simulink model "D_20231120_Modell_Inbetriebnahme_BreakOutBox_Jetson"  (R2022b)
(part 6 of 8)

  CAN Unpack94/16 -> Bus Creator94/7  "CAN ID"
  CAN Unpack94/17 -> Bus Creator94/8  "Timestamp"
  Bus Creator94/1 -> Bus Creator1/94  "Data_093"
  CAN Unpack94/1 -> Bus Creator94/1  "AZ_Winkel"
  CAN Unpack95/3 -> Terminator840/1
  CAN Unpack95/2 -> Bus Creator95/2  "EL_Angle"
  CAN Unpack95/13 -> Terminator847/1
  CAN Unpack95/7 -> Terminator844/1
  CAN Unpack95/12 -> Bus Creator95/5  "Range"
  CAN Unpack95/10 -> Bus Creator95/3  "Mode_Signal"
  CAN Unpack95/4 -> Terminator841/1
  CAN Unpack95/5 -> Terminator842/1
  CAN Unpack95/8 -> Terminator845/1
  CAN Unpack95/11 -> Bus Creator95/4  "RCS"
  CAN Unpack95/14 -> Terminator848/1
  CAN Unpack95/15 -> Bus Creator95/6  "Speed_Radial"
  CAN Unpack95/9 -> Terminator846/1
  CAN Unpack95/6 -> Terminator843/1
  CAN Unpack95/16 -> Bus Creator95/7  "CAN ID"
  CAN Unpack95/17 -> Bus Creator95/8  "Timestamp"
  Bus Creator95/1 -> Bus Creator1/95  "Data_094"
  CAN Unpack95/1 -> Bus Creator95/1  "AZ_Winkel"
  CAN Unpack96/3 -> Terminator849/1
  CAN Unpack96/2 -> Bus Creator96/2  "EL_Angle"
  CAN Unpack96/13 -> Terminator856/1
  CAN Unpack96/7 -> Terminator853/1
  CAN Unpack96/12 -> Bus Creator96/5  "Range"
  CAN Unpack96/10 -> Bus Creator96/3  "Mode_Signal"
  CAN Unpack96/4 -> Terminator850/1
  CAN Unpack96/5 -> Terminator851/1
  CAN Unpack96/8 -> Terminator854/1
  CAN Unpack96/11 -> Bus Creator96/4  "RCS"
  CAN Unpack96/14 -> Terminator857/1
  CAN Unpack96/15 -> Bus Creator96/6  "Speed_Radial"
  CAN Unpack96/9 -> Terminator855/1
  CAN Unpack96/6 -> Terminator852/1
  CAN Unpack96/16 -> Bus Creator96/7  "CAN ID"
  CAN Unpack96/17 -> Bus Creator96/8  "Timestamp"
  Bus Creator96/1 -> Bus Creator1/96  "Data_095"
  CAN Unpack96/1 -> Bus Creator96/1  "AZ_Winkel"
  CAN Unpack97/3 -> Terminator858/1
  CAN Unpack97/2 -> Bus Creator97/2  "EL_Angle"
  CAN Unpack97/13 -> Terminator865/1
  CAN Unpack97/7 -> Terminator862/1
  CAN Unpack97/12 -> Bus Creator97/5  "Range"
  CAN Unpack97/10 -> Bus Creator97/3  "Mode_Signal"
  CAN Unpack97/4 -> Terminator859/1
  CAN Unpack97/5 -> Terminator860/1
  CAN Unpack97/8 -> Terminator863/1
  CAN Unpack97/11 -> Bus Creator97/4  "RCS"
  CAN Unpack97/14 -> Terminator866/1
  CAN Unpack97/15 -> Bus Creator97/6  "Speed_Radial"
  CAN Unpack97/9 -> Terminator864/1
  CAN Unpack97/6 -> Terminator861/1
  CAN Unpack97/16 -> Bus Creator97/7  "CAN ID"
  CAN Unpack97/17 -> Bus Creator97/8  "Timestamp"
  Bus Creator97/1 -> Bus Creator1/97  "Data_096"
  CAN Unpack97/1 -> Bus Creator97/1  "AZ_Winkel"
  CAN Unpack98/3 -> Terminator867/1
  CAN Unpack98/2 -> Bus Creator98/2  "EL_Angle"
  CAN Unpack98/13 -> Terminator874/1
  CAN Unpack98/7 -> Terminator871/1
  CAN Unpack98/12 -> Bus Creator98/5  "Range"
  CAN Unpack98/10 -> Bus Creator98/3  "Mode_Signal"
  CAN Unpack98/4 -> Terminator868/1
  CAN Unpack98/5 -> Terminator869/1
  CAN Unpack98/8 -> Terminator872/1
  CAN Unpack98/11 -> Bus Creator98/4  "RCS"
  CAN Unpack98/14 -> Terminator875/1
  CAN Unpack98/15 -> Bus Creator98/6  "Speed_Radial"
  CAN Unpack98/9 -> Terminator873/1
  CAN Unpack98/6 -> Terminator870/1
  CAN Unpack98/16 -> Bus Creator98/7  "CAN ID"
  CAN Unpack98/17 -> Bus Creator98/8  "Timestamp"
  Bus Creator98/1 -> Bus Creator1/98  "Data_097"
  CAN Unpack98/1 -> Bus Creator98/1  "AZ_Winkel"
  CAN Unpack99/3 -> Terminator876/1
  CAN Unpack99/2 -> Bus Creator99/2  "EL_Angle"
  CAN Unpack99/13 -> Terminator883/1
  CAN Unpack99/7 -> Terminator880/1
  CAN Unpack99/12 -> Bus Creator99/5  "Range"
  CAN Unpack99/10 -> Bus Creator99/3  "Mode_Signal"
  CAN Unpack99/4 -> Terminator877/1
  CAN Unpack99/5 -> Terminator878/1
  CAN Unpack99/8 -> Terminator881/1
  CAN Unpack99/11 -> Bus Creator99/4  "RCS"
  CAN Unpack99/14 -> Terminator884/1
  CAN Unpack99/15 -> Bus Creator99/6  "Speed_Radial"
  CAN Unpack99/9 -> Terminator882/1
  CAN Unpack99/6 -> Terminator879/1
  CAN Unpack99/16 -> Bus Creator99/7  "CAN ID"
  CAN Unpack99/17 -> Bus Creator99/8  "Timestamp"
  Bus Creator99/1 -> Bus Creator1/99  "Data_098"
  CAN Unpack99/1 -> Bus Creator99/1  "AZ_Winkel"
  CAN Unpack100/3 -> Terminator885/1
  CAN Unpack100/2 -> Bus Creator100/2  "EL_Angle"
  CAN Unpack100/13 -> Terminator892/1
  CAN Unpack100/7 -> Terminator889/1
  CAN Unpack100/12 -> Bus Creator100/5  "Range"
  CAN Unpack100/10 -> Bus Creator100/3  "Mode_Signal"
  CAN Unpack100/4 -> Terminator886/1
  CAN Unpack100/5 -> Terminator887/1
  CAN Unpack100/8 -> Terminator890/1
  CAN Unpack100/11 -> Bus Creator100/4  "RCS"
  CAN Unpack100/14 -> Terminator893/1
  CAN Unpack100/15 -> Bus Creator100/6  "Speed_Radial"
  CAN Unpack100/9 -> Terminator891/1
  CAN Unpack100/6 -> Terminator888/1
  CAN Unpack100/16 -> Bus Creator100/7  "CAN ID"
  CAN Unpack100/17 -> Bus Creator100/8  "Timestamp"
  Bus Creator100/1 -> Bus Creator1/100  "Data_099"
  CAN Unpack100/1 -> Bus Creator100/1  "AZ_Winkel"
  CAN Unpack101/3 -> Terminator894/1
  CAN Unpack101/2 -> Bus Creator101/2  "EL_Angle"
  CAN Unpack101/13 -> Terminator901/1
  CAN Unpack101/7 -> Terminator898/1
  CAN Unpack101/12 -> Bus Creator101/5  "Range"
  CAN Unpack101/10 -> Bus Creator101/3  "Mode_Signal"
  CAN Unpack101/4 -> Terminator895/1
  CAN Unpack101/5 -> Terminator896/1
  CAN Unpack101/8 -> Terminator899/1
  CAN Unpack101/11 -> Bus Creator101/4  "RCS"
  CAN Unpack101/14 -> Terminator902/1
  CAN Unpack101/15 -> Bus Creator101/6  "Speed_Radial"
  CAN Unpack101/9 -> Terminator900/1
  CAN Unpack101/6 -> Terminator897/1
  CAN Unpack101/16 -> Bus Creator101/7  "CAN ID"
  CAN Unpack101/17 -> Bus Creator101/8  "Timestamp"
  Bus Creator101/1 -> Bus Creator1/101  "Data_100"
  CAN Unpack101/1 -> Bus Creator101/1  "AZ_Winkel"
  CAN Unpack102/3 -> Terminator903/1
  CAN Unpack102/2 -> Bus Creator102/2  "EL_Angle"
  CAN Unpack102/13 -> Terminator910/1
  CAN Unpack102/7 -> Terminator907/1
  CAN Unpack102/12 -> Bus Creator102/5  "Range"
  CAN Unpack102/10 -> Bus Creator102/3  "Mode_Signal"
  CAN Unpack102/4 -> Terminator904/1
  CAN Unpack102/5 -> Terminator905/1
  CAN Unpack102/8 -> Terminator908/1
  CAN Unpack102/11 -> Bus Creator102/4  "RCS"
  CAN Unpack102/14 -> Terminator911/1
  CAN Unpack102/15 -> Bus Creator102/6  "Speed_Radial"
  CAN Unpack102/9 -> Terminator909/1
  CAN Unpack102/6 -> Terminator906/1
  CAN Unpack102/16 -> Bus Creator102/7  "CAN ID"
  CAN Unpack102/17 -> Bus Creator102/8  "Timestamp"
  Bus Creator102/1 -> Bus Creator1/102  "Data_101"
  CAN Unpack102/1 -> Bus Creator102/1  "AZ_Winkel"
  CAN Unpack103/3 -> Terminator912/1
  CAN Unpack103/2 -> Bus Creator103/2  "EL_Angle"
  CAN Unpack103/13 -> Terminator919/1
  CAN Unpack103/7 -> Terminator916/1
  CAN Unpack103/12 -> Bus Creator103/5  "Range"
  CAN Unpack103/10 -> Bus Creator103/3  "Mode_Signal"
  CAN Unpack103/4 -> Terminator913/1
  CAN Unpack103/5 -> Terminator914/1
  CAN Unpack103/8 -> Terminator917/1
  CAN Unpack103/11 -> Bus Creator103/4  "RCS"
  CAN Unpack103/14 -> Terminator920/1
  CAN Unpack103/15 -> Bus Creator103/6  "Speed_Radial"
  CAN Unpack103/9 -> Terminator918/1
  CAN Unpack103/6 -> Terminator915/1
  CAN Unpack103/16 -> Bus Creator103/7  "CAN ID"
  CAN Unpack103/17 -> Bus Creator103/8  "Timestamp"
  Bus Creator103/1 -> Bus Creator1/103  "Data_102"
  CAN Unpack103/1 -> Bus Creator103/1  "AZ_Winkel"
  CAN Unpack104/3 -> Terminator921/1
  CAN Unpack104/2 -> Bus Creator104/2  "EL_Angle"
  CAN Unpack104/13 -> Terminator928/1
  CAN Unpack104/7 -> Terminator925/1
  CAN Unpack104/12 -> Bus Creator104/5  "Range"
  CAN Unpack104/10 -> Bus Creator104/3  "Mode_Signal"
  CAN Unpack104/4 -> Terminator922/1
  CAN Unpack104/5 -> Terminator923/1
  CAN Unpack104/8 -> Terminator926/1
  CAN Unpack104/11 -> Bus Creator104/4  "RCS"
  CAN Unpack104/14 -> Terminator929/1
  CAN Unpack104/15 -> Bus Creator104/6  "Speed_Radial"
  CAN Unpack104/9 -> Terminator927/1
  CAN Unpack104/6 -> Terminator924/1
  CAN Unpack104/16 -> Bus Creator104/7  "CAN ID"
  CAN Unpack104/17 -> Bus Creator104/8  "Timestamp"
  Bus Creator104/1 -> Bus Creator1/104  "Data_103"
  CAN Unpack104/1 -> Bus Creator104/1  "AZ_Winkel"
  CAN Unpack105/3 -> Terminator930/1
  CAN Unpack105/2 -> Bus Creator105/2  "EL_Angle"
  CAN Unpack105/13 -> Terminator937/1
  CAN Unpack105/7 -> Terminator934/1
  CAN Unpack105/12 -> Bus Creator105/5  "Range"
  CAN Unpack105/10 -> Bus Creator105/3  "Mode_Signal"
  CAN Unpack105/4 -> Terminator931/1
  CAN Unpack105/5 -> Terminator932/1
  CAN Unpack105/8 -> Terminator935/1
  CAN Unpack105/11 -> Bus Creator105/4  "RCS"
  CAN Unpack105/14 -> Terminator938/1
  CAN Unpack105/15 -> Bus Creator105/6  "Speed_Radial"
  CAN Unpack105/9 -> Terminator936/1
  CAN Unpack105/6 -> Terminator933/1
  CAN Unpack105/16 -> Bus Creator105/7  "CAN ID"
  CAN Unpack105/17 -> Bus Creator105/8  "Timestamp"
  Bus Creator105/1 -> Bus Creator1/105  "Data_104"
  CAN Unpack105/1 -> Bus Creator105/1  "AZ_Winkel"
  CAN Unpack106/3 -> Terminator939/1
  CAN Unpack106/2 -> Bus Creator106/2  "EL_Angle"
  CAN Unpack106/13 -> Terminator946/1
  CAN Unpack106/7 -> Terminator943/1
  CAN Unpack106/12 -> Bus Creator106/5  "Range"
  CAN Unpack106/10 -> Bus Creator106/3  "Mode_Signal"
  CAN Unpack106/4 -> Terminator940/1
  CAN Unpack106/5 -> Terminator941/1
  CAN Unpack106/8 -> Terminator944/1
  CAN Unpack106/11 -> Bus Creator106/4  "RCS"
  CAN Unpack106/14 -> Terminator947/1
  CAN Unpack106/15 -> Bus Creator106/6  "Speed_Radial"
  CAN Unpack106/9 -> Terminator945/1
  CAN Unpack106/6 -> Terminator942/1
  CAN Unpack106/16 -> Bus Creator106/7  "CAN ID"
  CAN Unpack106/17 -> Bus Creator106/8  "Timestamp"
  Bus Creator106/1 -> Bus Creator1/106  "Data_105"
  CAN Unpack106/1 -> Bus Creator106/1  "AZ_Winkel"
  CAN Unpack107/3 -> Terminator948/1
  CAN Unpack107/2 -> Bus Creator107/2  "EL_Angle"
  CAN Unpack107/13 -> Terminator955/1
  CAN Unpack107/7 -> Terminator952/1
  CAN Unpack107/12 -> Bus Creator107/5  "Range"
  CAN Unpack107/10 -> Bus Creator107/3  "Mode_Signal"
  CAN Unpack107/4 -> Terminator949/1
  CAN Unpack107/5 -> Terminator950/1
  CAN Unpack107/8 -> Terminator953/1
  CAN Unpack107/11 -> Bus Creator107/4  "RCS"
  CAN Unpack107/14 -> Terminator956/1
  CAN Unpack107/15 -> Bus Creator107/6  "Speed_Radial"
  CAN Unpack107/9 -> Terminator954/1
  CAN Unpack107/6 -> Terminator951/1
  CAN Unpack107/16 -> Bus Creator107/7  "CAN ID"
  CAN Unpack107/17 -> Bus Creator107/8  "Timestamp"
  Bus Creator107/1 -> Bus Creator1/107  "Data_106"
  CAN Unpack107/1 -> Bus Creator107/1  "AZ_Winkel"
  CAN Unpack108/3 -> Terminator957/1
  CAN Unpack108/2 -> Bus Creator108/2  "EL_Angle"
  CAN Unpack108/13 -> Terminator964/1
  CAN Unpack108/7 -> Terminator961/1
  CAN Unpack108/12 -> Bus Creator108/5  "Range"
  CAN Unpack108/10 -> Bus Creator108/3  "Mode_Signal"
  CAN Unpack108/4 -> Terminator958/1
  CAN Unpack108/5 -> Terminator959/1
  CAN Unpack108/8 -> Terminator962/1
  CAN Unpack108/11 -> Bus Creator108/4  "RCS"
  CAN Unpack108/14 -> Terminator965/1
  CAN Unpack108/15 -> Bus Creator108/6  "Speed_Radial"
  CAN Unpack108/9 -> Terminator963/1
  CAN Unpack108/6 -> Terminator960/1
  CAN Unpack108/16 -> Bus Creator108/7  "CAN ID"
  CAN Unpack108/17 -> Bus Creator108/8  "Timestamp"
  Bus Creator108/1 -> Bus Creator1/108  "Data_107"
  CAN Unpack108/1 -> Bus Creator108/1  "AZ_Winkel"
  CAN Unpack109/3 -> Terminator966/1
  CAN Unpack109/2 -> Bus Creator109/2  "EL_Angle"
  CAN Unpack109/13 -> Terminator973/1
  CAN Unpack109/7 -> Terminator970/1
  CAN Unpack109/12 -> Bus Creator109/5  "Range"
  CAN Unpack109/10 -> Bus Creator109/3  "Mode_Signal"
  CAN Unpack109/4 -> Terminator967/1
  CAN Unpack109/5 -> Terminator968/1
  CAN Unpack109/8 -> Terminator971/1
  CAN Unpack109/11 -> Bus Creator109/4  "RCS"
  CAN Unpack109/14 -> Terminator974/1
  CAN Unpack109/15 -> Bus Creator109/6  "Speed_Radial"
  CAN Unpack109/9 -> Terminator972/1
  CAN Unpack109/6 -> Terminator969/1
  CAN Unpack109/16 -> Bus Creator109/7  "CAN ID"
  CAN Unpack109/17 -> Bus Creator109/8  "Timestamp"
  Bus Creator109/1 -> Bus Creator1/109  "Data_108"
  CAN Unpack109/1 -> Bus Creator109/1  "AZ_Winkel"
  CAN Unpack110/3 -> Terminator975/1
  CAN Unpack110/2 -> Bus Creator110/2  "EL_Angle"
  CAN Unpack110/13 -> Terminator982/1
  CAN Unpack110/7 -> Terminator979/1
  CAN Unpack110/12 -> Bus Creator110/5  "Range"
  CAN Unpack110/10 -> Bus Creator110/3  "Mode_Signal"
  CAN Unpack110/4 -> Terminator976/1
  CAN Unpack110/5 -> Terminator977/1
  CAN Unpack110/8 -> Terminator980/1
  CAN Unpack110/11 -> Bus Creator110/4  "RCS"
  CAN Unpack110/14 -> Terminator983/1
  CAN Unpack110/15 -> Bus Creator110/6  "Speed_Radial"
  CAN Unpack110/9 -> Terminator981/1
  CAN Unpack110/6 -> Terminator978/1
  CAN Unpack110/16 -> Bus Creator110/7  "CAN ID"
  CAN Unpack110/17 -> Bus Creator110/8  "Timestamp"
  Bus Creator110/1 -> Bus Creator1/110  "Data_109"
  CAN Unpack110/1 -> Bus Creator110/1  "AZ_Winkel"
  CAN Unpack111/3 -> Terminator984/1
  CAN Unpack111/2 -> Bus Creator111/2  "EL_Angle"
  CAN Unpack111/13 -> Terminator991/1
  CAN Unpack111/7 -> Terminator988/1
  CAN Unpack111/12 -> Bus Creator111/5  "Range"
  CAN Unpack111/10 -> Bus Creator111/3  "Mode_Signal"
  CAN Unpack111/4 -> Terminator985/1
  CAN Unpack111/5 -> Terminator986/1
  CAN Unpack111/8 -> Terminator989/1
  CAN Unpack111/11 -> Bus Creator111/4  "RCS"
  CAN Unpack111/14 -> Terminator992/1
  CAN Unpack111/15 -> Bus Creator111/6  "Speed_Radial"
  CAN Unpack111/9 -> Terminator990/1
  CAN Unpack111/6 -> Terminator987/1
  CAN Unpack111/16 -> Bus Creator111/7  "CAN ID"
  CAN Unpack111/17 -> Bus Creator111/8  "Timestamp"
  Bus Creator111/1 -> Bus Creator1/111  "Data_110"
  CAN Unpack111/1 -> Bus Creator111/1  "AZ_Winkel"
  CAN Unpack112/3 -> Terminator993/1
  CAN Unpack112/2 -> Bus Creator112/2  "EL_Angle"
  CAN Unpack112/13 -> Terminator1000/1
  CAN Unpack112/7 -> Terminator997/1
  CAN Unpack112/12 -> Bus Creator112/5  "Range"
  CAN Unpack112/10 -> Bus Creator112/3  "Mode_Signal"
  CAN Unpack112/4 -> Terminator994/1
  CAN Unpack112/5 -> Terminator995/1
  CAN Unpack112/8 -> Terminator998/1
  CAN Unpack112/11 -> Bus Creator112/4  "RCS"
  CAN Unpack112/14 -> Terminator1001/1
  CAN Unpack112/15 -> Bus Creator112/6  "Speed_Radial"
  CAN Unpack112/9 -> Terminator999/1
  CAN Unpack112/6 -> Terminator996/1
  CAN Unpack112/16 -> Bus Creator112/7  "CAN ID"
  CAN Unpack112/17 -> Bus Creator112/8  "Timestamp"
  Bus Creator112/1 -> Bus Creator1/112  "Data_111"
  CAN Unpack112/1 -> Bus Creator112/1  "AZ_Winkel"
  CAN Unpack113/3 -> Terminator1002/1
  CAN Unpack113/2 -> Bus Creator113/2  "EL_Angle"
  CAN Unpack113/13 -> Terminator1009/1
  CAN Unpack113/7 -> Terminator1006/1
  CAN Unpack113/12 -> Bus Creator113/5  "Range"
  CAN Unpack113/10 -> Bus Creator113/3  "Mode_Signal"
  CAN Unpack113/4 -> Terminator1003/1
  CAN Unpack113/5 -> Terminator1004/1
  CAN Unpack113/8 -> Terminator1007/1
  CAN Unpack113/11 -> Bus Creator113/4  "RCS"
  CAN Unpack113/14 -> Terminator1010/1
  CAN Unpack113/15 -> Bus Creator113/6  "Speed_Radial"
  CAN Unpack113/9 -> Terminator1008/1
  CAN Unpack113/6 -> Terminator1005/1
  CAN Unpack113/16 -> Bus Creator113/7  "CAN ID"
  CAN Unpack113/17 -> Bus Creator113/8  "Timestamp"
  Bus Creator113/1 -> Bus Creator1/113  "Data_112"
  CAN Unpack113/1 -> Bus Creator113/1  "AZ_Winkel"
  CAN Unpack114/3 -> Terminator1011/1
  CAN Unpack114/2 -> Bus Creator114/2  "EL_Angle"
  CAN Unpack114/13 -> Terminator1018/1
  CAN Unpack114/7 -> Terminator1015/1
  CAN Unpack114/12 -> Bus Creator114/5  "Range"
  CAN Unpack114/10 -> Bus Creator114/3  "Mode_Signal"
  CAN Unpack114/4 -> Terminator1012/1
  CAN Unpack114/5 -> Terminator1013/1
  CAN Unpack114/8 -> Terminator1016/1
  CAN Unpack114/11 -> Bus Creator114/4  "RCS"
  CAN Unpack114/14 -> Terminator1019/1
  CAN Unpack114/15 -> Bus Creator114/6  "Speed_Radial"
  CAN Unpack114/9 -> Terminator1017/1
  CAN Unpack114/6 -> Terminator1014/1
  CAN Unpack114/16 -> Bus Creator114/7  "CAN ID"
  CAN Unpack114/17 -> Bus Creator114/8  "Timestamp"
  Bus Creator114/1 -> Bus Creator1/114  "Data_113"
  CAN Unpack114/1 -> Bus Creator114/1  "AZ_Winkel"
  CAN Unpack115/3 -> Terminator1020/1
  CAN Unpack115/2 -> Bus Creator115/2  "EL_Angle"
  CAN Unpack115/13 -> Terminator1027/1
  CAN Unpack115/7 -> Terminator1024/1
  CAN Unpack115/12 -> Bus Creator115/5  "Range"
  CAN Unpack115/10 -> Bus Creator115/3  "Mode_Signal"
  CAN Unpack115/4 -> Terminator1021/1
  CAN Unpack115/5 -> Terminator1022/1
  CAN Unpack115/8 -> Terminator1025/1
  CAN Unpack115/11 -> Bus Creator115/4  "RCS"
  CAN Unpack115/14 -> Terminator1028/1
  CAN Unpack115/15 -> Bus Creator115/6  "Speed_Radial"
  CAN Unpack115/9 -> Terminator1026/1
  CAN Unpack115/6 -> Terminator1023/1
  CAN Unpack115/16 -> Bus Creator115/7  "CAN ID"
  CAN Unpack115/17 -> Bus Creator115/8  "Timestamp"
  Bus Creator115/1 -> Bus Creator1/115  "Data_114"
  CAN Unpack115/1 -> Bus Creator115/1  "AZ_Winkel"
  CAN Unpack116/3 -> Terminator1029/1
  CAN Unpack116/2 -> Bus Creator116/2  "EL_Angle"
  CAN Unpack116/13 -> Terminator1036/1
  CAN Unpack116/7 -> Terminator1033/1
  CAN Unpack116/12 -> Bus Creator116/5  "Range"
  CAN Unpack116/10 -> Bus Creator116/3  "Mode_Signal"
  CAN Unpack116/4 -> Terminator1030/1
  CAN Unpack116/5 -> Terminator1031/1
  CAN Unpack116/8 -> Terminator1034/1
  CAN Unpack116/11 -> Bus Creator116/4  "RCS"
  CAN Unpack116/14 -> Terminator1037/1
  CAN Unpack116/15 -> Bus Creator116/6  "Speed_Radial"
  CAN Unpack116/9 -> Terminator1035/1
  CAN Unpack116/6 -> Terminator1032/1
  CAN Unpack116/16 -> Bus Creator116/7  "CAN ID"
  CAN Unpack116/17 -> Bus Creator116/8  "Timestamp"
  Bus Creator116/1 -> Bus Creator1/116  "Data_115"
  CAN Unpack116/1 -> Bus Creator116/1  "AZ_Winkel"
  CAN Unpack117/3 -> Terminator1038/1
  CAN Unpack117/2 -> Bus Creator117/2  "EL_Angle"
  CAN Unpack117/13 -> Terminator1045/1
  CAN Unpack117/7 -> Terminator1042/1
  CAN Unpack117/12 -> Bus Creator117/5  "Range"
  CAN Unpack117/10 -> Bus Creator117/3  "Mode_Signal"
  CAN Unpack117/4 -> Terminator1039/1
  CAN Unpack117/5 -> Terminator1040/1
  CAN Unpack117/8 -> Terminator1043/1
  CAN Unpack117/11 -> Bus Creator117/4  "RCS"
  CAN Unpack117/14 -> Terminator1046/1
  CAN Unpack117/15 -> Bus Creator117/6  "Speed_Radial"
  CAN Unpack117/9 -> Terminator1044/1
  CAN Unpack117/6 -> Terminator1041/1
  CAN Unpack117/16 -> Bus Creator117/7  "CAN ID"
  CAN Unpack117/17 -> Bus Creator117/8  "Timestamp"
  Bus Creator117/1 -> Bus Creator1/117  "Data_116"
  CAN Unpack117/1 -> Bus Creator117/1  "AZ_Winkel"
  CAN Unpack118/3 -> Terminator1047/1
  CAN Unpack118/2 -> Bus Creator118/2  "EL_Angle"
  CAN Unpack118/13 -> Terminator1054/1
  CAN Unpack118/7 -> Terminator1051/1
  CAN Unpack118/12 -> Bus Creator118/5  "Range"
  CAN Unpack118/10 -> Bus Creator118/3  "Mode_Signal"
  CAN Unpack118/4 -> Terminator1048/1
  CAN Unpack118/5 -> Terminator1049/1
  CAN Unpack118/8 -> Terminator1052/1
  CAN Unpack118/11 -> Bus Creator118/4  "RCS"
  CAN Unpack118/14 -> Terminator1055/1
  CAN Unpack118/15 -> Bus Creator118/6  "Speed_Radial"
  CAN Unpack118/9 -> Terminator1053/1
  CAN Unpack118/6 -> Terminator1050/1
  CAN Unpack118/16 -> Bus Creator118/7  "CAN ID"
  CAN Unpack118/17 -> Bus Creator118/8  "Timestamp"
  Bus Creator118/1 -> Bus Creator1/118  "Data_117"
  CAN Unpack118/1 -> Bus Creator118/1  "AZ_Winkel"
  CAN Unpack119/3 -> Terminator1056/1
  CAN Unpack119/2 -> Bus Creator119/2  "EL_Angle"
  CAN Unpack119/13 -> Terminator1063/1
  CAN Unpack119/7 -> Terminator1060/1
  CAN Unpack119/12 -> Bus Creator119/5  "Range"
  CAN Unpack119/10 -> Bus Creator119/3  "Mode_Signal"
  CAN Unpack119/4 -> Terminator1057/1
  CAN Unpack119/5 -> Terminator1058/1
  CAN Unpack119/8 -> Terminator1061/1
  CAN Unpack119/11 -> Bus Creator119/4  "RCS"
  CAN Unpack119/14 -> Terminator1064/1
  CAN Unpack119/15 -> Bus Creator119/6  "Speed_Radial"
  CAN Unpack119/9 -> Terminator1062/1
  CAN Unpack119/6 -> Terminator1059/1
  CAN Unpack119/16 -> Bus Creator119/7  "CAN ID"
  CAN Unpack119/17 -> Bus Creator119/8  "Timestamp"
  Bus Creator119/1 -> Bus Creator1/119  "Data_118"
  CAN Unpack119/1 -> Bus Creator119/1  "AZ_Winkel"
  CAN Unpack120/3 -> Terminator1065/1
  CAN Unpack120/2 -> Bus Creator120/2  "EL_Angle"
  CAN Unpack120/13 -> Terminator1072/1
  CAN Unpack120/7 -> Terminator1069/1
  CAN Unpack120/12 -> Bus Creator120/5  "Range"
  CAN Unpack120/10 -> Bus Creator120/3  "Mode_Signal"
  CAN Unpack120/4 -> Terminator1066/1
  CAN Unpack120/5 -> Terminator1067/1
  CAN Unpack120/8 -> Terminator1070/1
  CAN Unpack120/11 -> Bus Creator120/4  "RCS"
  CAN Unpack120/14 -> Terminator1073/1
  CAN Unpack120/15 -> Bus Creator120/6  "Speed_Radial"
  CAN Unpack120/9 -> Terminator1071/1
  CAN Unpack120/6 -> Terminator1068/1
  CAN Unpack120/16 -> Bus Creator120/7  "CAN ID"
  CAN Unpack120/17 -> Bus Creator120/8  "Timestamp"
  Bus Creator120/1 -> Bus Creator1/120  "Data_119"
  CAN Unpack120/1 -> Bus Creator120/1  "AZ_Winkel"
  CAN Unpack121/3 -> Terminator1074/1
  CAN Unpack121/2 -> Bus Creator121/2  "EL_Angle"
  CAN Unpack121/13 -> Terminator1081/1
  CAN Unpack121/7 -> Terminator1078/1
  CAN Unpack121/12 -> Bus Creator121/5  "Range"
  CAN Unpack121/10 -> Bus Creator121/3  "Mode_Signal"
  CAN Unpack121/4 -> Terminator1075/1
  CAN Unpack121/5 -> Terminator1076/1
  CAN Unpack121/8 -> Terminator1079/1
  CAN Unpack121/11 -> Bus Creator121/4  "RCS"
  CAN Unpack121/14 -> Terminator1082/1
  CAN Unpack121/15 -> Bus Creator121/6  "Speed_Radial"
  CAN Unpack121/9 -> Terminator1080/1
  CAN Unpack121/6 -> Terminator1077/1
  CAN Unpack121/16 -> Bus Creator121/7  "CAN ID"
  CAN Unpack121/17 -> Bus Creator121/8  "Timestamp"
  Bus Creator121/1 -> Bus Creator1/121  "Data_120"
  CAN Unpack121/1 -> Bus Creator121/1  "AZ_Winkel"
  CAN Unpack122/3 -> Terminator1083/1
  CAN Unpack122/2 -> Bus Creator122/2  "EL_Angle"
  CAN Unpack122/13 -> Terminator1090/1
  CAN Unpack122/7 -> Terminator1087/1
  CAN Unpack122/12 -> Bus Creator122/5  "Range"
  CAN Unpack122/10 -> Bus Creator122/3  "Mode_Signal"
  CAN Unpack122/4 -> Terminator1084/1
  CAN Unpack122/5 -> Terminator1085/1
  CAN Unpack122/8 -> Terminator1088/1
  CAN Unpack122/11 -> Bus Creator122/4  "RCS"
  CAN Unpack122/14 -> Terminator1091/1
  CAN Unpack122/15 -> Bus Creator122/6  "Speed_Radial"
  CAN Unpack122/9 -> Terminator1089/1
  CAN Unpack122/6 -> Terminator1086/1
  CAN Unpack122/16 -> Bus Creator122/7  "CAN ID"
  CAN Unpack122/17 -> Bus Creator122/8  "Timestamp"
  Bus Creator122/1 -> Bus Creator1/122  "Data_121"
  CAN Unpack122/1 -> Bus Creator122/1  "AZ_Winkel"
  CAN Unpack123/3 -> Terminator1092/1
  CAN Unpack123/2 -> Bus Creator123/2  "EL_Angle"
  CAN Unpack123/13 -> Terminator1099/1
  CAN Unpack123/7 -> Terminator1096/1
  CAN Unpack123/12 -> Bus Creator123/5  "Range"
  CAN Unpack123/10 -> Bus Creator123/3  "Mode_Signal"
  CAN Unpack123/4 -> Terminator1093/1
  CAN Unpack123/5 -> Terminator1094/1
  CAN Unpack123/8 -> Terminator1097/1
  CAN Unpack123/11 -> Bus Creator123/4  "RCS"
  CAN Unpack123/14 -> Terminator1100/1
  CAN Unpack123/15 -> Bus Creator123/6  "Speed_Radial"
  CAN Unpack123/9 -> Terminator1098/1
  CAN Unpack123/6 -> Terminator1095/1
  CAN Unpack123/16 -> Bus Creator123/7  "CAN ID"
  CAN Unpack123/17 -> Bus Creator123/8  "Timestamp"
  Bus Creator123/1 -> Bus Creator1/123  "Data_122"
  CAN Unpack123/1 -> Bus Creator123/1  "AZ_Winkel"
  CAN Unpack124/3 -> Terminator1101/1
  CAN Unpack124/2 -> Bus Creator124/2  "EL_Angle"
  CAN Unpack124/13 -> Terminator1108/1
  CAN Unpack124/7 -> Terminator1105/1
  CAN Unpack124/12 -> Bus Creator124/5  "Range"
  CAN Unpack124/10 -> Bus Creator124/3  "Mode_Signal"
  CAN Unpack124/4 -> Terminator1102/1
  CAN Unpack124/5 -> Terminator1103/1
  CAN Unpack124/8 -> Terminator1106/1
  CAN Unpack124/11 -> Bus Creator124/4  "RCS"
  CAN Unpack124/14 -> Terminator1109/1
  CAN Unpack124/15 -> Bus Creator124/6  "Speed_Radial"
  CAN Unpack124/9 -> Terminator1107/1
  CAN Unpack124/6 -> Terminator1104/1
  CAN Unpack124/16 -> Bus Creator124/7  "CAN ID"
  CAN Unpack124/17 -> Bus Creator124/8  "Timestamp"
  Bus Creator124/1 -> Bus Creator1/124  "Data_123"
  CAN Unpack124/1 -> Bus Creator124/1  "AZ_Winkel"
  CAN Unpack125/3 -> Terminator1110/1
  CAN Unpack125/2 -> Bus Creator125/2  "EL_Angle"
  CAN Unpack125/13 -> Terminator1117/1
  CAN Unpack125/7 -> Terminator1114/1
  CAN Unpack125/12 -> Bus Creator125/5  "Range"
  CAN Unpack125/10 -> Bus Creator125/3  "Mode_Signal"
  CAN Unpack125/4 -> Terminator1111/1
  CAN Unpack125/5 -> Terminator1112/1
  CAN Unpack125/8 -> Terminator1115/1
  CAN Unpack125/11 -> Bus Creator125/4  "RCS"
  CAN Unpack125/14 -> Terminator1118/1
  CAN Unpack125/15 -> Bus Creator125/6  "Speed_Radial"
  CAN Unpack125/9 -> Terminator1116/1
  CAN Unpack125/6 -> Terminator1113/1
  CAN Unpack125/16 -> Bus Creator125/7  "CAN ID"
  CAN Unpack125/17 -> Bus Creator125/8  "Timestamp"
  Bus Creator125/1 -> Bus Creator1/125  "Data_124"
  CAN Unpack125/1 -> Bus Creator125/1  "AZ_Winkel"
  CAN Unpack126/3 -> Terminator1119/1
  CAN Unpack126/2 -> Bus Creator126/2  "EL_Angle"
  CAN Unpack126/13 -> Terminator1126/1
  CAN Unpack126/7 -> Terminator1123/1
  CAN Unpack126/12 -> Bus Creator126/5  "Range"
  CAN Unpack126/10 -> Bus Creator126/3  "Mode_Signal"
  CAN Unpack126/4 -> Terminator1120/1
  CAN Unpack126/5 -> Terminator1121/1
  CAN Unpack126/8 -> Terminator1124/1
  CAN Unpack126/11 -> Bus Creator126/4  "RCS"
  CAN Unpack126/14 -> Terminator1127/1
  CAN Unpack126/15 -> Bus Creator126/6  "Speed_Radial"
  CAN Unpack126/9 -> Terminator1125/1
  CAN Unpack126/6 -> Terminator1122/1
  CAN Unpack126/16 -> Bus Creator126/7  "CAN ID"
  CAN Unpack126/17 -> Bus Creator126/8  "Timestamp"
  Bus Creator126/1 -> Bus Creator1/126  "Data_125"
  CAN Unpack126/1 -> Bus Creator126/1  "AZ_Winkel"
  CAN Unpack127/3 -> Terminator1128/1
  CAN Unpack127/2 -> Bus Creator127/2  "EL_Angle"
  CAN Unpack127/13 -> Terminator1135/1
  CAN Unpack127/7 -> Terminator1132/1
  CAN Unpack127/12 -> Bus Creator127/5  "Range"
  CAN Unpack127/10 -> Bus Creator127/3  "Mode_Signal"
  CAN Unpack127/4 -> Terminator1129/1
  CAN Unpack127/5 -> Terminator1130/1
  CAN Unpack127/8 -> Terminator1133/1
  CAN Unpack127/11 -> Bus Creator127/4  "RCS"
  CAN Unpack127/14 -> Terminator1136/1
  CAN Unpack127/15 -> Bus Creator127/6  "Speed_Radial"
  CAN Unpack127/9 -> Terminator1134/1
  CAN Unpack127/6 -> Terminator1131/1
  CAN Unpack127/16 -> Bus Creator127/7  "CAN ID"
  CAN Unpack127/17 -> Bus Creator127/8  "Timestamp"
  Bus Creator127/1 -> Bus Creator1/127  "Data_126"
  CAN Unpack127/1 -> Bus Creator127/1  "AZ_Winkel"
  CAN Unpack128/3 -> Terminator1137/1
  CAN Unpack128/2 -> Bus Creator128/2  "EL_Angle"
  CAN Unpack128/13 -> Terminator1144/1
  CAN Unpack128/7 -> Terminator1141/1
  CAN Unpack128/12 -> Bus Creator128/5  "Range"
  CAN Unpack128/10 -> Bus Creator128/3  "Mode_Signal"
  CAN Unpack128/4 -> Terminator1138/1
  CAN Unpack128/5 -> Terminator1139/1
  CAN Unpack128/8 -> Terminator1142/1
  CAN Unpack128/11 -> Bus Creator128/4  "RCS"
  CAN Unpack128/14 -> Terminator1145/1
  CAN Unpack128/15 -> Bus Creator128/6  "Speed_Radial"
  CAN Unpack128/9 -> Terminator1143/1
  CAN Unpack128/6 -> Terminator1140/1
  CAN Unpack128/16 -> Bus Creator128/7  "CAN ID"
  CAN Unpack128/17 -> Bus Creator128/8  "Timestamp"
  Bus Creator128/1 -> Bus Creator1/128  "Data_127"
  CAN Unpack128/1 -> Bus Creator128/1  "AZ_Winkel"
  CAN Unpack129/3 -> Terminator1146/1
  CAN Unpack129/2 -> Bus Creator129/2  "EL_Angle"
  CAN Unpack129/13 -> Terminator1153/1
  CAN Unpack129/7 -> Terminator1150/1
  CAN Unpack129/12 -> Bus Creator129/5  "Range"
  CAN Unpack129/10 -> Bus Creator129/3  "Mode_Signal"
  CAN Unpack129/4 -> Terminator1147/1
  CAN Unpack129/5 -> Terminator1148/1
  CAN Unpack129/8 -> Terminator1151/1
  CAN Unpack129/11 -> Bus Creator129/4  "RCS"
  CAN Unpack129/14 -> Terminator1154/1
  CAN Unpack129/15 -> Bus Creator129/6  "Speed_Radial"
  CAN Unpack129/9 -> Terminator1152/1
  CAN Unpack129/6 -> Terminator1149/1
  CAN Unpack129/16 -> Bus Creator129/7  "CAN ID"
  CAN Unpack129/17 -> Bus Creator129/8  "Timestamp"
  Bus Creator129/1 -> Bus Creator1/129  "Data_128"
  CAN Unpack129/1 -> Bus Creator129/1  "AZ_Winkel"
